simulink model "PI"  (R2020b)
settings: Solver=VariableStepAuto  StartTime=0.0  StopTime=10  RelTol=1e-3
values from neighbouring files (symbols this model uses):
  Ki = 65    [IntializePara.m]    (also in matlab_Cruise.mat)
  Kp = 1200    [IntializePara.m]    (also in matlab_Cruise.mat)
settings Model: Creator=BIDITA PAUL  LastModifiedBy=BIDITA PAUL
settings DataIOCC: SaveOutput=off  SaveTime=off

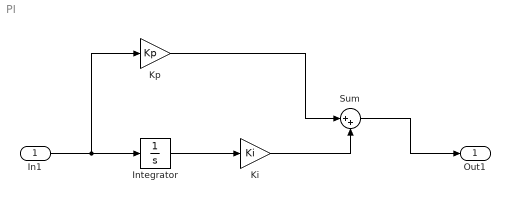
== system PI ==
  In1 : Inport  OutDataTypeStr=double  PortDimensions=1  SampleTime=0
  Integrator : Integrator
  Ki : Gain  Gain=Ki
  Kp : Gain  Gain=Kp
  Sum : Sum  Inputs=|++
  Out1 : Outport  OutDataTypeStr=double  PortDimensions=1  SampleTime=0
  wires:
  Kp/1 -> Sum/1
  Ki/1 -> Sum/2
  Integrator/1 -> Ki/1
  In1/1 -> Kp/1, Integrator/1
  Sum/1 -> Out1/1
